simulink model "mech_car_handling"  (Simulink 7.1)
settings: Solver=ode15s  StartTime=0.0  StopTime=150  RelTol=1e-3
PostLoadFcn:
  | %%%%%%%%%%%%%%%%%%%%%%%%%%%%%%%%%%%%%%%%%%%%%%%%%%%%%%%%%%%%%%%%%%%%%%%%%%%
  | % INITIALIZE VEHICLE PARAMETERS
  | %%%%%%%%%%%%%%%%%%%%%%%%%%%%%%%%%%%%%%%%%%%%%%%%%%%%%%%%%%%%%%%%%%%%%%%%%%%
  | %clear;
  | %echo on;
  | 
  | % INITIALIZE STRUCTURES
  | chassis = struct();
  | wheel = struct();
  | axle = struct();
  | 
  | % INITIALIZE CHASSIS PARAMETERS
  | chassis.a = 1.50;          % longitudinal distance from CG to front axle
  | chassis.b = 0.99;           % longitudinal distance from CG to rear axle
  | chassis.w = 0.9;           % chassis width (wheel to wheel distance)
  | chassis.hu = 0.1;          % height of unsprung mass above ground
  | chassis.hs = 0.3;          % height of sprung mass above unsprung mass
  | chassis.ms = 1470;      % mass of sprung mass
  | chassis.mu = 200;        % mass of unsprung mass
  | 
  | % INITIALIZE WHEEL PARAMETERS
  | wheel.r = 0.3;             % wheel radius
  | wheel.m = 30;            % wheel mass
  | wheel.I = [0.52 0 0;0 1 0;0 0 0.52];
  | 
  | % INITIALIZE AXLE PARAMETERS
  | axle.m = 2;                 % axle mass
  | 
  | % COMPUTE STEADY STATE LOADS
  | Fzf = 0.5*(chassis.ms+chassis.mu) * 9.81 * chassis.b / (chassis.a + chassis.b);    % initial front wheel reaction
  | Fzr = 0.5*(chassis.ms+chassis.mu) * 9.81 * chassis. a / (chassis.a + chassis.b);    % initial rear wheel reaction
  | 
  | % INITIALIZE ROLL PARAMETERS
  | kf = 9000;                 % sprung front roll stiffness
  | kb = 5500;                % sprung rear roll stiffness
  | ku = 10000;              % unsprung roll stiffness (same front and rear)
  | bu = 0.1 * ku;            % unsprung roll damping
  | kr = kf + kb;              % total sprung roll stiffness
  | br = 0.1*kr;                % sprung roll damping
  | 
  | % INITIALIZE NONLINEAR TIRE MODEL PARAMETERS
  | a1 = 1.8658e-5;            % nonlinear tire model proportional coefficient
  | a2 = 9.3290e-4;            % nonlinear tire model quadratic coefficient
  | 
  | % INITIALIZE CONTROLLER PARAMETERS
  | Kp = 10000;                 % speed controller proportional gain
  | 
  | % INITIALIZE STEERING PARAMETERS
  | steeringAngle = 2;
  | %echo off;
StopFcn:
  | appDataName = 'mech_car_steering_fig_data';
  | mech_car_handling_fig_mgr('init',appDataName);
  | 
  | p = size(speed.signals.values);
  | p = p(1);
  | R = speed.signals.values([30:p])./yaw_rate.signals.values([30:p]);
  | modelFigure = getappdata(0,'mech_car_steering_fig_data');
  | plot(speed.signals.values([30:p]),R,'g','Parent',modelFigure.axesH);
libraries: mblibv1 x33, simulink x3
(part 1 of 2)
Description:
  | Car Handling
  | 
  | This model simulates the handling of a car for a set of chassis, wheel and axle characteristics. You can simulate the model for one roll stiffness, or for a range of roll stiffnesses by clicking on the blue subsystem.
  | 
  | The model shows that when a car is accelerated at a constant steering angle, it circles either out or in, depending on whether the car is understeered or oversteered, respectively.
CloseFcn:
  | appDataName = 'mech_car_steering_fig_data';
  | mech_car_handling_fig_mgr('destroy',appDataName);
settings Model: Creator=arnav  LastModifiedBy=batserve  ExtModeAutoUpdateStatusClock=off
settings DebuggingCC: SaveWithParameterizedLinksMsg=none  SignalResolutionControl=TryResolveAllWithWarning  SolverPrmCheckMsg=none  MultiTaskDSMMsg=warning  MultiTaskCondExecSysMsg=none  StrictBusMsg=None
settings HardwareCC: TargetBitPerLong=64  TargetEndianess=LittleEndian  TargetWordSize=64  TargetHWDeviceType=MATLAB Host  ProdEqTarget=off
settings RTWCC: SystemTargetFile=rsim.tlc  TemplateMakefile=rsim_default_tmf  Description=Rapid Simulation Target  ProcessScript=rsim_make_rtw_hook  IncludeERTFirstTime=on
settings RSimTargetCC: TargetFcnLib=ansi_tfl_tmw.mat  TargetFunctionLibrary=ANSI_C  IsPILTarget=off  EnableShiftOperators=on  PortableWordSizes=off
settings SimMechanicsCC: WarnOnRedundantConstraints=off

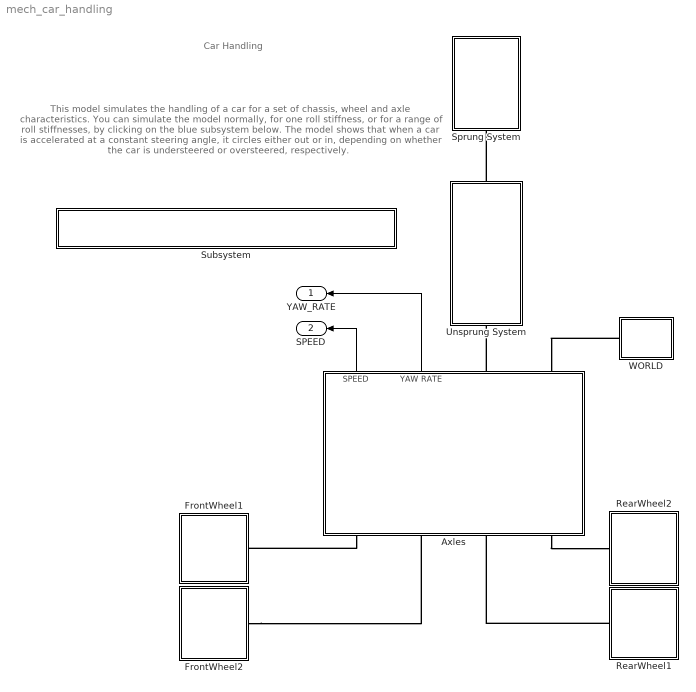
== system mech_car_handling ==
  note: Car Handling
  note: This model simulates the handling of a car for
      | a set of chassis, wheel and axle characteristics.
      | You can simulate the model normally, for one roll stiffness, or
      | for a range of roll stiffnesses, by clicking on the blue subsystem below.
      |
      | The model shows that when a car is accelerated at a constant steering
      | angle, it circles either out or in, depending on whether
      | the car is understeered or oversteered, respectively.
  Axles : Subsystem  Orientation=up  mask{w=chassis.w, a=chassis.a, b=chassis.b, m=axle.m}
      mask prompts: w "Axle Length"; a "CG to Front Axle Distance"; b "CG to Rear Axle Distance"; m "Axle Mass"
      mask Display: image(imread('double_wishbone.jpg'))
  FrontWheel1 : Subsystem  Orientation=left
      mask Display: image(imread('wheel.jpg'))
  FrontWheel2 : Subsystem  Orientation=left
      mask Display: image(imread('wheel.jpg'))
  RearWheel1 : Subsystem
      mask Display: image(imread('wheel.jpg'))
  RearWheel2 : Subsystem
      mask Display: image(imread('wheel.jpg'))
  Sprung System : Subsystem  Orientation=up
  Subsystem : Subsystem
      settings: OpenFcn=mech_car_handling_sweep
      mask Display: disp('CLICK HERE TO RUN FOR A RANGE OF ROLL STIFFNESSES')
  Unsprung System : Subsystem  Orientation=up
  WORLD : Subsystem
      mask Display: image(imread('sky.jpg'))
  YAW_RATE : Outport  Orientation=left  OutDataType=sfix(16)  OutScaling=2^0
  SPEED : Outport  Orientation=left  Port=2  OutDataType=sfix(16)  OutScaling=2^0
  wires:
  Axles/1(SPEED) -> SPEED/1
  Axles/2(YAW RATE) -> YAW_RATE/1
  connections:
  WORLD/LConn1 -- Axles/RConn2
  FrontWheel2/LConn1 -- Axles/LConn2
  RearWheel1/LConn1 -- Axles/LConn3
  Axles/LConn4 -- RearWheel2/LConn1
  Axles/LConn1 -- FrontWheel1/LConn1
  Axles/RConn1 -- Unsprung System/LConn1
  Unsprung System/RConn1 -- Sprung System/LConn1

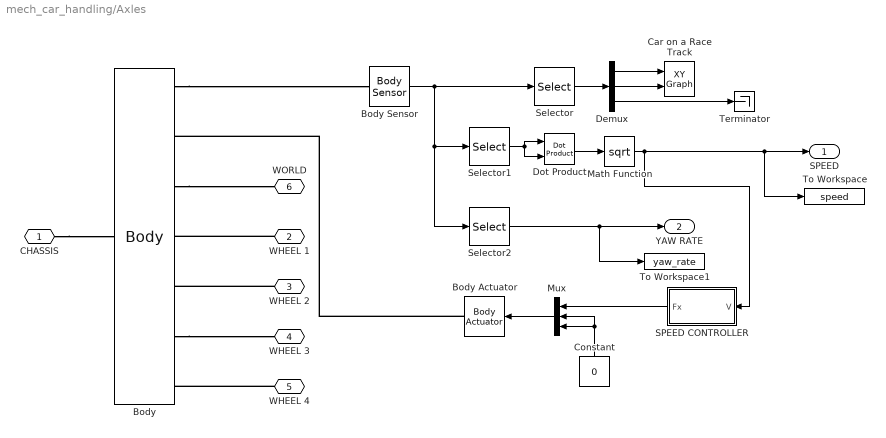
== system mech_car_handling/Axles ==
  Body : mblibv1/Bodies/Body  DialogController=MECH.DynMechDlgSource  PhysicalDomain=mechanical  SubClassName=Unknown  LeftPortType=workingframe  RightPortType=workingframe  LConnTagsString=CG  RConnTagsString=CS6|CS7|CS3|CS1|CS2|CS4|CS5  DialogClass=MechanicalBodyBlock  Mass=2*m  MassUnits=kg  InertiaUnits=kg*m^2  Inertia=[0.12 0 0; 0 1.5 0;0 0 1.5]  Shape=Cylinder  ShapeDims=[1 1]  ShapeUnits=m  ShapeUse=false  Density=1  DensityUnits=kg/m^3  DensityUse=false  GraphicsMode=1  BodyColor=[0.5 0.5 0.5]  GraphicsObj=[]  AttachedToCS=1  CG=Left$CG$[0 0 0]$CS3$CS3$m$[0 0 0]$EULER X-Y-Z$deg$WORLD$true  WorkingFrames=Right$CS6$[0 0 0]$CS3$CS3$m$[0 0 0]$EULER X-Y-Z$deg$WORLD$true#Right$CS7$[0 0 0]$CS3$CS3$m$[0 0 0]$EULER X-Y-Z$deg$WORLD$true#Right$CS3$[0 0 0]$ADJOINING$ADJOINING$m$[0 0 0]$EULER X-Y-Z$deg$WORLD$true#Right$CS1$[a -0.5*w 0]$CS3$CS3$m$[0 0 0]$EULER X-Y-Z$deg$WORLD$true#Right$CS2$[a 0.5*w 0]$CS3$CS3$m$[0 0 0]$EULER X-Y-Z$deg$WORLD$true#Right$CS4$[-b -0.5*w 0]$CS3$CS3$m$[0 0 0]$EULER X-Y-Z$deg$WORLD$true#Right$CS5$[-b 0.5*w 0]$CS3$CS3$m$[0 0 0]$EULER X-Y-Z$deg$WORLD$true  CGPos=[0 0 0]  CGRot=[0 0 0]  CS0Pos=[]  CS0Rot=[]  CS1Pos=[a -0.5*w 0]  CS1Rot=[0 0 0]  CS2Pos=[a 0.5*w 0]  CS2Rot=[0 0 0]  CS3Pos=[0 0 0]  CS3Rot=[0 0 0]  CS4Pos=[-b -0.5*w 0]  CS4Rot=[0 0 0]  CS5Pos=[-b 0.5*w 0]  CS5Rot=[0 0 0]  CS6Pos=[0 0 0]  CS6Rot=[0 0 0]  CS7Pos=[0 0 0]  CS7Rot=[0 0 0]  CS8Pos=[]  CS8Rot=[]  CS9Pos=[]  CS9Rot=[]  CS10Pos=[]  CS10Rot=[]  CS11Pos=[]  CS11Rot=[]  CS12Pos=[]  CS12Rot=[]  CS13Pos=[]  CS13Rot=[]  CS14Pos=[]  CS14Rot=[]  CS15Pos=[]  CS15Rot=[]  CS16Pos=[]  CS16Rot=[]  CS17Pos=[]  CS17Rot=[]  CS18Pos=[]  CS18Rot=[]  CS19Pos=[]  CS19Rot=[]  CS20Pos=[]  CS20Rot=[]
  Body Actuator : mblibv1/Sensors &  Actuators/Body Actuator  Orientation=left  DialogController=MECH.DynMechDlgSource  SystemSampleTime=-1  PhysicalDomain=Mechanical  PortType=blob  ActuationStyle=Force  AngleUnits=deg  ArcVelocityUnits=deg/s  ArcAccelerationUnits=deg/s^2  CoordPositionUnits=m  VelocityUnits=m/s  AccelerationUnits=m/s^2  ForceUnits=N  TorqueUnits=N-m  ActiveIO=on  Width=3  DialogClass=MechanicalActuatorBlock  ReferenceFrame=Local (Body CS)  Angle=off  CoordPosition=on  Force=on  Torque=off
  Body Sensor : mblibv1/Sensors &  Actuators/Body Sensor  DialogController=MECH.DynMechDlgSource  SystemSampleTime=-1  PhysicalDomain=Mechanical  PortType=blob  Muxed=on  Pose=off  Angle=on  AngleUnits=deg  ArcVelocity=on  ArcVelocityUnits=rad/s  ArcAcceleration=off  ArcAccelerationUnits=deg/s^2  CoordPosition=on  CoordPositionUnits=m  Velocity=on  VelocityUnits=m/s  Acceleration=off  AccelerationUnits=m/s^2  Quaternion=on  QuaternionDT=off  QuaternionDDT=off  QuaternionUnits=off  OutputVector=[ 3 3 3 ]  ActiveIO=on  Width=9  DialogClass=MechanicalSensorBlock  ReferenceFrame=Absolute (World)
  Car on a Race Track : simulink/Sinks/XY Graph  SystemSampleTime=-1  xmin=-200  xmax=200  ymin=-100  ymax=250  st=-1
  Constant : Constant  Orientation=up  Value=0  OutDataType=sfix(16)  OutScaling=2^0
  Demux : Demux  Outputs=3
  Dot Product : simulink/Math Operations/Dot Product  InputSameDT=on  OutDataType=sfix(16)  OutScaling=2^-10  DoSatur=off
  Math Function : Math  Operator=sqrt  OutDataType=sfix(16)  OutScaling=2^0  SaturateOnIntegerOverflow=on
  Mux : Mux  Orientation=left  Inputs=3
  SPEED CONTROLLER : Subsystem  Orientation=left
  Selector : Selector  InputPortWidth=9  IndexOptions=Index vector (dialog)  Indices=[1 2 3]  OutputSizes=1
  Selector1 : Selector  InputPortWidth=9  IndexOptions=Index vector (dialog)  Indices=[4 5]  OutputSizes=1
  Selector2 : Selector  InputPortWidth=9  IndexOptions=Index vector (dialog)  Indices=9  OutputSizes=1
  Terminator : Terminator
  To Workspace : ToWorkspace  VariableName=speed  SampleTime=-1  SaveFormat=Structure
  To Workspace1 : ToWorkspace  VariableName=yaw_rate  SampleTime=-1  SaveFormat=Structure
  CHASSIS : PMIOPort  Port=1  Side=Right
  WHEEL 1 : PMIOPort  Orientation=left  Port=2  Side=Left
  WHEEL 2 : PMIOPort  Orientation=left  Port=3  Side=Left
  WHEEL 3 : PMIOPort  Orientation=left  Port=4  Side=Left
  WHEEL 4 : PMIOPort  Orientation=left  Port=5  Side=Left
  WORLD : PMIOPort  Orientation=left  Port=6  Side=Right
  SPEED : Outport  OutDataType=sfix(16)  OutScaling=2^0
  YAW RATE : Outport  Port=2  OutDataType=sfix(16)  OutScaling=2^0
  wires:
  Demux/1 -> Car on a Race Track/1
  Demux/2 -> Car on a Race Track/2
  Dot Product/1 -> Math Function/1
  Math Function/1 -> SPEED CONTROLLER/1(V), SPEED/1, To Workspace/1
  Selector/1 -> Demux/1
  Body Sensor/1 -> Selector/1, Selector1/1, Selector2/1
  Selector1/1 -> Dot Product/1, Dot Product/2
  Selector2/1 -> YAW RATE/1, To Workspace1/1
  Constant/1 -> Mux/3, Mux/2
  Mux/1 -> Body Actuator/1
  SPEED CONTROLLER/1(Fx) -> Mux/1
  Demux/3 -> Terminator/1
  connections:
  WHEEL 1/RConn1 -- Body/RConn4
  CHASSIS/RConn1 -- Body/LConn1
  WHEEL 2/RConn1 -- Body/RConn5
  Body/RConn3 -- WORLD/RConn1
  WHEEL 4/RConn1 -- Body/RConn7
  Body/RConn6 -- WHEEL 3/RConn1
  Body/RConn1 -- Body Sensor/LConn1
  Body Actuator/RConn1 -- Body/RConn2

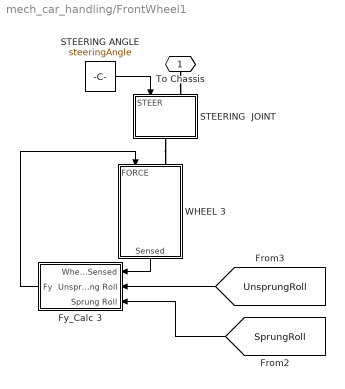
== system mech_car_handling/FrontWheel1 ==
  Fy_Calc 3 : Subsystem  Orientation=left
  STEERING ANGLE : Constant  Value=steeringAngle  OutDataType=sfix(16)  OutScaling=2^0
  STEERING  JOINT : Subsystem  Orientation=down
  WHEEL 3 : Subsystem  Orientation=down  mask{r=wheel.r, m=wheel.m, I=wheel.I}
      mask prompts: r "Wheel Radius"; m "Wheel Mass"; I "Wheel Inertia"
  To Chassis : PMIOPort  Orientation=down  Port=1  Side=Left
  wires:
  STEERING ANGLE/1 -> STEERING  JOINT/1(STEER)
  Fy_Calc 3/1(Fy) -> WHEEL 3/1(FORCE)
  WHEEL 3/1(Sensed) -> Fy_Calc 3/1(Wheel Sensed)
  [UnsprungRoll] -> Fy_Calc 3/2(Unsprung Roll)
  [SprungRoll] -> Fy_Calc 3/3(Sprung Roll)
  connections:
  STEERING  JOINT/RConn1 -- WHEEL 3/LConn1
  To Chassis/RConn1 -- STEERING  JOINT/LConn1

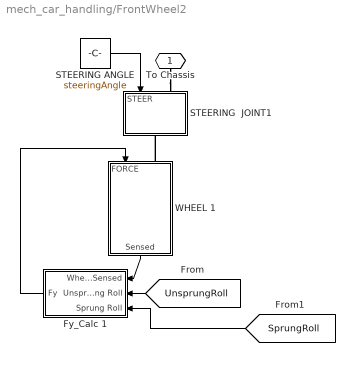
== system mech_car_handling/FrontWheel2 ==
  Fy_Calc 1 : Subsystem  Orientation=left
  STEERING ANGLE : Constant  Value=steeringAngle  OutDataType=sfix(16)  OutScaling=2^0
  STEERING  JOINT1 : Subsystem  Orientation=down
  WHEEL 1 : Subsystem  Orientation=down  mask{r=wheel.r, m=wheel.m, I=wheel.I}
      mask prompts: r "Wheel Radius"; m "Wheel Mass"; I "Wheel Inertia"
  To Chassis : PMIOPort  Orientation=down  Port=1  Side=Left
  wires:
  WHEEL 1/1(Sensed) -> Fy_Calc 1/1(Wheel Sensed)
  [UnsprungRoll] -> Fy_Calc 1/2(Unsprung Roll)
  [SprungRoll] -> Fy_Calc 1/3(Sprung Roll)
  STEERING ANGLE/1 -> STEERING  JOINT1/1(STEER)
  Fy_Calc 1/1(Fy) -> WHEEL 1/1(FORCE)
  connections:
  WHEEL 1/LConn1 -- STEERING  JOINT1/RConn1
  To Chassis/RConn1 -- STEERING  JOINT1/LConn1

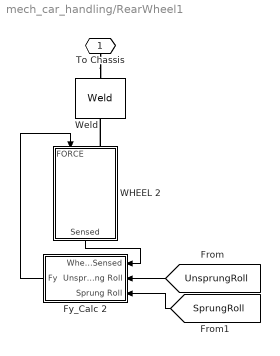
== system mech_car_handling/RearWheel1 ==
  Fy_Calc 2 : Subsystem  Orientation=left
  WHEEL 2 : Subsystem  Orientation=down  mask{r=wheel.r, m=wheel.m, I=wheel.I}
      mask prompts: r "Wheel Radius"; m "Wheel Mass"; I "Wheel Inertia"
  Weld : mblibv1/Joints/Weld  Orientation=down  DialogController=MECH.DynMechDlgSource  PhysicalDomain=mechanical  SubClassName=Unknown  LeftPortType=blob  RightPortType=blob  LConnTagsString=__newl0  RConnTagsString=__newr0  NumSAPorts=0  CutJoint=off  MarkAsCut=off  Primitives=weld  PrimitiveProps=W$INERTIAL$[0 0 0]$weld  DialogClass=JointBlock  WAxis=[0 0 0]
  To Chassis : PMIOPort  Orientation=down  Port=1  Side=Left
  wires:
  Fy_Calc 2/1(Fy) -> WHEEL 2/1(FORCE)
  WHEEL 2/1(Sensed) -> Fy_Calc 2/1(Wheel Sensed)
  [UnsprungRoll] -> Fy_Calc 2/2(Unsprung Roll)
  [SprungRoll] -> Fy_Calc 2/3(Sprung Roll)
  connections:
  WHEEL 2/LConn1 -- Weld/RConn1
  To Chassis/RConn1 -- Weld/LConn1

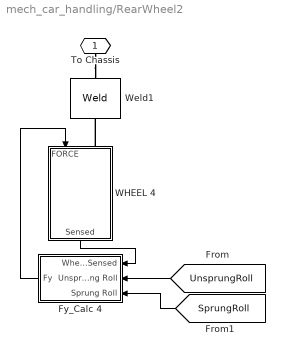
== system mech_car_handling/RearWheel2 ==
  Fy_Calc 4 : Subsystem  Orientation=left
  WHEEL 4 : Subsystem  Orientation=down  mask{r=wheel.r, m=wheel.m, I=wheel.I}
      mask prompts: r "Wheel Radius"; m "Wheel Mass"; I "Wheel Inertia"
  Weld1 : mblibv1/Joints/Weld  Orientation=down  DialogController=MECH.DynMechDlgSource  PhysicalDomain=mechanical  SubClassName=Unknown  LeftPortType=blob  RightPortType=blob  LConnTagsString=__newl0  RConnTagsString=__newr0  NumSAPorts=0  CutJoint=off  MarkAsCut=off  Primitives=weld  PrimitiveProps=W$INERTIAL$[0 0 0]$weld  DialogClass=JointBlock  WAxis=[0 0 0]
  To Chassis : PMIOPort  Orientation=down  Port=1  Side=Left
  wires:
  Fy_Calc 4/1(Fy) -> WHEEL 4/1(FORCE)
  WHEEL 4/1(Sensed) -> Fy_Calc 4/1(Wheel Sensed)
  [UnsprungRoll] -> Fy_Calc 4/2(Unsprung Roll)
  [SprungRoll] -> Fy_Calc 4/3(Sprung Roll)
  connections:
  WHEEL 4/LConn1 -- Weld1/RConn1
  To Chassis/RConn1 -- Weld1/LConn1

== system mech_car_handling/Sprung System ==
  note: Sprung mass represents the
      | total mass of the car: the mass
      | of the wheels and chassis.
  SPRUNG MASS : Subsystem  Orientation=down  mask{a=chassis.a, b=chassis.b, m=chassis.ms, h=chassis.hs}
      mask prompts: a "Front Axle to CG Distance"; b "Rear Axle to CG Distance"; m "Chassis Mass"; h "CG Height (above axles)"
  TORSIONAL SPRING1 : Subsystem  Orientation=up
  To UnSprungMass : PMIOPort  Orientation=up  Port=1  Side=Left
  tag scope: SprungRoll=global
  wires:
  TORSIONAL SPRING1/1(Roll) -> [SprungRoll]
  connections:
  TORSIONAL SPRING1/RConn1 -- SPRUNG MASS/RConn1
  To UnSprungMass/RConn1 -- TORSIONAL SPRING1/LConn1

== system mech_car_handling/Subsystem ==

== system mech_car_handling/Unsprung System ==
  note: Sprung mass represents the
      | the mass of the wheels and
      | chassis only.
  TORSIONAL SPRING : Subsystem  Orientation=up
  UNSPRUNG MASS : Subsystem  Orientation=down  mask{a=chassis.a, b=chassis.b, m=chassis.mu, h=chassis.hu}
      mask prompts: a "Front Axle to CG Distance"; b "Rear Axle to CG Distance"; m "Chassis Mass"; h "CG Height (above axles)"
  To SprungSystem : PMIOPort  Orientation=down  Port=1  Side=Right
  To Chassis : PMIOPort  Orientation=up  Port=2  Side=Left
  tag scope: UnsprungRoll=global
  wires:
  TORSIONAL SPRING/1(Roll) -> [UnsprungRoll]
  connections:
  TORSIONAL SPRING/RConn1 -- UNSPRUNG MASS/RConn1
  To SprungSystem/RConn1 -- UNSPRUNG MASS/LConn1
  To Chassis/RConn1 -- TORSIONAL SPRING/LConn1

== system mech_car_handling/WORLD ==
  Ground : mblibv1/Bodies/Ground  Orientation=left  DialogController=MECH.DynMechDlgSource  SystemSampleTime=-1  LeftPortType=env  RightPortType=workingframe  PhysicalDomain=Mechanical  DialogClass=GroundBlock  CoordPosition=[0 0 0]  CoordPositionUnits=m  StateVectorMgrId=-1  MachineId=[0 0]  ShowEnvPort=on
  Joint Initial Condition : mblibv1/Sensors &  Actuators/Joint Initial Condition  DialogController=MECH.DynMechDlgSource  SystemSampleTime=-1  PhysicalDomain=mechanical  DialogClass=InitialConditionBlock  InitialConditions=P1$true$0$m$rad$2$m/s$rad/s#P2$true$0$m$rad$0$m/s$rad/s#P3$false$0$m$rad$0$m/s$rad/s#R1$false$0$m$rad$0$m/s$rad/s#R2$false$0$m$rad$0$m/s$rad/s#R3$false$0$m$rad$0$m/s$rad/s#S$false$0$m$rad$0$m/s$rad/s  P1PIC=0  P1VIC=2  P2PIC=0  P2VIC=0  P3PIC=0  P3VIC=0  R1PIC=0  R1VIC=0  R2PIC=0  R2VIC=0  R3PIC=0  R3VIC=0  SPIC=0  SVIC=0
  Machine Environment : mblibv1/Bodies/Machine Environment  Tag=Factory ground  Orientation=left  DialogController=MECH.DialogSource  SystemSampleTime=-1  PortType=env  PhysicalDomain=Mechanical  DialogTemplateClass=MECH.MachineEnvironment  SyncWhenCopied=off  Gravity=[0 0 -9.81]  GravityUnits=m/s^2  GravityAsSignal=off  Dimensionality=Auto-detect  AnalysisType=Forward dynamics  LinearAssemblyTolerance=1e-3  LinearAssemblyToleranceUnits=m  AngularAssemblyTolerance=1e-3  AngularAssemblyToleranceUnits=rad  ConstraintSolverType=Stabilizing  ConstraintRelTolerance=1e-4  ConstraintAbsTolerance=1e-4  UseRobustSingularityHandling=off  RedundancyAnalysisToleranceType=Automatically select tolerance  RedundancyAnalysisTolerance=1e-14  StatePerturbationType=Fixed  PerturbationSize=1e-5  VisualizeMachine=on
  Planar : mblibv1/Joints/Planar  Orientation=left  DialogController=MECH.DynMechDlgSource  PhysicalDomain=mechanical  SubClassName=Unknown  LeftPortType=blob  RightPortType=blob  LConnTagsString=__newl0|SA1  RConnTagsString=__newr0  NumSAPorts=1  CutJoint=off  MarkAsCut=off  Primitives=prismatic_prismatic_revolute  PrimitiveProps=P1$WORLD$[1 0 0]$prismatic#P2$WORLD$[0 1 0]$prismatic#R1$WORLD$[0 0 1]$revolute  DialogClass=JointBlock  P1Axis=[1 0 0]  P2Axis=[0 1 0]  R1Axis=[0 0 1]
  F : PMIOPort  Port=1  Side=Left
  connections:
  Machine Environment/RConn1 -- Ground/LConn1
  F/RConn1 -- Planar/RConn1
  Ground/RConn1 -- Planar/LConn1
  Joint Initial Condition/RConn1 -- Planar/LConn2

== system mech_car_handling/Axles/SPEED CONTROLLER ==
  V : Inport  OutDataType=sfix(16)  OutScaling=2^0
  Kp : Gain  Gain=Kp  ParameterDataType=sfix(16)  ParameterScaling=2^0  OutDataType=sfix(16)  OutScaling=2^0
  Kp1 : Gain  Gain=-1  ParameterDataType=sfix(16)  ParameterScaling=2^0  OutDataType=sfix(16)  OutScaling=2^0
  Ramp : simulink/Sources/Ramp  SystemSampleTime=-1  slope=0.1  start=0  X0=5
  Subtract2 : Sum  Inputs=+-  OutDataType=sfix(16)  OutScaling=2^-10
  Fx : Outport  OutDataType=sfix(16)  OutScaling=2^0
  wires:
  V/1 -> Subtract2/1
  Subtract2/1 -> Kp/1
  Ramp/1 -> Subtract2/2
  Kp1/1 -> Fx/1
  Kp/1 -> Kp1/1

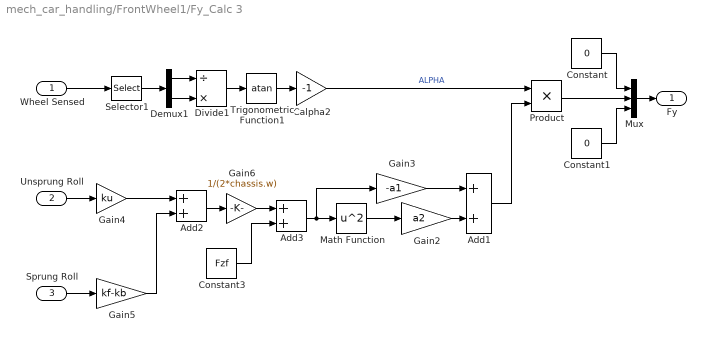
== system mech_car_handling/FrontWheel1/Fy_Calc 3 ==
  Wheel Sensed : Inport  OutDataType=sfix(16)  OutScaling=2^0
  Unsprung Roll : Inport  Port=2  OutDataType=sfix(16)  OutScaling=2^0
  Sprung Roll : Inport  Port=3  OutDataType=sfix(16)  OutScaling=2^0
  Add1 : Sum  OutDataType=sfix(16)  OutScaling=2^-10
  Add2 : Sum  OutDataType=sfix(16)  OutScaling=2^-10
  Add3 : Sum  OutDataType=sfix(16)  OutScaling=2^-10
  Calpha2 : Gain  Gain=-1  ParameterDataType=sfix(16)  ParameterScaling=2^0  OutDataType=sfix(16)  OutScaling=2^0
  Constant : Constant  Value=0  OutDataType=sfix(16)  OutScaling=2^0
  Constant1 : Constant  Value=0  OutDataType=sfix(16)  OutScaling=2^0
  Constant3 : Constant  Value=Fzf  OutDataType=sfix(16)  OutScaling=2^0
  Demux1 : Demux  Outputs=2
  Divide1 : Product  Inputs=/*  OutDataType=sfix(16)  OutScaling=2^-10
  Gain2 : Gain  Gain=a2  ParameterDataType=sfix(16)  ParameterScaling=2^0  OutDataType=sfix(16)  OutScaling=2^0
  Gain3 : Gain  Gain=-a1  ParameterDataType=sfix(16)  ParameterScaling=2^0  OutDataType=sfix(16)  OutScaling=2^0
  Gain4 : Gain  Gain=ku  ParameterDataType=sfix(16)  ParameterScaling=2^0  OutDataType=sfix(16)  OutScaling=2^0
  Gain5 : Gain  Gain=kf-kb  ParameterDataType=sfix(16)  ParameterScaling=2^0  OutDataType=sfix(16)  OutScaling=2^0
  Gain6 : Gain  Gain=1/(2*chassis.w)  ParameterDataType=sfix(16)  ParameterScaling=2^0  OutDataType=sfix(16)  OutScaling=2^0
  Math Function : Math  Operator=square  OutDataType=sfix(16)  OutScaling=2^0  SaturateOnIntegerOverflow=on
  Mux : Mux  Inputs=3
  Product : Product  OutDataType=sfix(16)  OutScaling=2^0  RndMeth=Zero
  Selector1 : Selector  InputPortWidth=3  IndexOptions=Index vector (dialog)  Indices=[1 2]  OutputSizes=1
  Trigonometric Function1 : Trigonometry  Operator=atan
  Fy : Outport  OutDataType=sfix(16)  OutScaling=2^0
  wires:
  Calpha2/1 -> Product/1  "ALPHA"
  Divide1/1 -> Trigonometric Function1/1
  Demux1/2 -> Divide1/2
  Demux1/1 -> Divide1/1
  Selector1/1 -> Demux1/1
  Constant1/1 -> Mux/3
  Constant/1 -> Mux/1
  Mux/1 -> Fy/1
  Product/1 -> Mux/2
  Wheel Sensed/1 -> Selector1/1
  Trigonometric Function1/1 -> Calpha2/1
  Math Function/1 -> Gain2/1
  Gain2/1 -> Add1/2
  Gain3/1 -> Add1/1
  Add1/1 -> Product/2
  Unsprung Roll/1 -> Gain4/1
  Sprung Roll/1 -> Gain5/1
  Gain4/1 -> Add2/1
  Gain5/1 -> Add2/2
  Add2/1 -> Gain6/1
  Gain6/1 -> Add3/1
  Constant3/1 -> Add3/2
  Add3/1 -> Math Function/1, Gain3/1

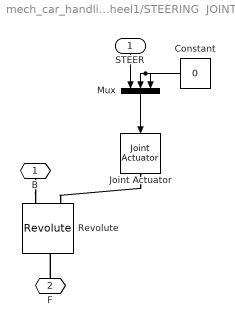
== system mech_car_handling/FrontWheel1/STEERING  JOINT ==
  STEER : Inport  Orientation=down  OutDataType=sfix(16)  OutScaling=2^0
  Constant : Constant  Orientation=left  Value=0  OutDataType=sfix(16)  OutScaling=2^0
  Joint Actuator : mblibv1/Sensors &  Actuators/Joint Actuator  Orientation=down  DialogController=MECH.DynMechDlgSource  SystemSampleTime=-1  PhysicalDomain=Mechanical  PortType=blob  ActuationStyle=Motion  AngleUnits=deg  ArcVelocityUnits=deg/s  ArcAccelerationUnits=deg/s^2  CoordPositionUnits=m  VelocityUnits=m/s  AccelerationUnits=m/s^2  ForceUnits=N  TorqueUnits=N-m  ActiveIO=on  Width=3  DialogClass=MechanicalActuatorBlock  Primitive=R1  ReferenceFrame=Absolute (INERTIAL)
  Mux : Mux  Orientation=down  Inputs=3
  Revolute : mblibv1/Joints/Revolute  Orientation=down  DialogController=MECH.DynMechDlgSource  PhysicalDomain=mechanical  SubClassName=Unknown  LeftPortType=blob  RightPortType=blob  LConnTagsString=__newl0|SA1  RConnTagsString=__newr0  NumSAPorts=1  CutJoint=off  MarkAsCut=off  Primitives=revolute  PrimitiveProps=R1$WORLD$[0 0 1]$revolute  DialogClass=JointBlock  R1Axis=[0 0 1]
  B : PMIOPort  Orientation=down  Port=1  Side=Left
  F : PMIOPort  Orientation=up  Port=2  Side=Right
  wires:
  STEER/1 -> Mux/1
  Mux/1 -> Joint Actuator/1
  Constant/1 -> Mux/2, Mux/3
  connections:
  Joint Actuator/RConn1 -- Revolute/LConn2
  B/RConn1 -- Revolute/LConn1
  F/RConn1 -- Revolute/RConn1

== system mech_car_handling/FrontWheel1/WHEEL 3 ==
  FORCE : Inport  Orientation=left  OutDataType=sfix(16)  OutScaling=2^0
  Body : mblibv1/Bodies/Body  DialogController=MECH.DynMechDlgSource  PhysicalDomain=mechanical  SubClassName=Unknown  LeftPortType=workingframe  RightPortType=workingframe  LConnTagsString=CG  RConnTagsString=CS2|CS3  DialogClass=MechanicalBodyBlock  Mass=m  MassUnits=kg  InertiaUnits=kg*m^2  Inertia=I  Shape=Cylinder  ShapeDims=[1 1]  ShapeUnits=m  ShapeUse=false  Density=1  DensityUnits=kg/m^3  DensityUse=false  GraphicsMode=1  BodyColor=[0.5 0.5 0.5]  GraphicsObj=[]  AttachedToCS=1  CG=Left$CG$[0 0 0]$ADJOINING$ADJOINING$m$[0 0 0]$EULER X-Y-Z$deg$WORLD$true  WorkingFrames=Right$CS2$[0 0 -r]$CG$CG$m$[0 0 0]$EULER X-Y-Z$deg$WORLD$true#Left$CS1$[0 0 -r]$CG$CG$m$[0 0 0]$EULER X-Y-Z$deg$WORLD$false#Right$CS3$[0 0 -r]$CG$CG$m$[0 0 0]$EULER X-Y-Z$deg$WORLD$true  CGPos=[0 0 0]  CGRot=[0 0 0]  CS0Pos=[]  CS0Rot=[]  CS1Pos=[0 0 -r]  CS1Rot=[0 0 0]  CS2Pos=[0 0 -r]  CS2Rot=[0 0 0]  CS3Pos=[0 0 -r]  CS3Rot=[0 0 0]  CS4Pos=[]  CS4Rot=[]  CS5Pos=[]  CS5Rot=[]  CS6Pos=[]  CS6Rot=[]  CS7Pos=[]  CS7Rot=[]  CS8Pos=[]  CS8Rot=[]  CS9Pos=[]  CS9Rot=[]  CS10Pos=[]  CS10Rot=[]  CS11Pos=[]  CS11Rot=[]  CS12Pos=[]  CS12Rot=[]  CS13Pos=[]  CS13Rot=[]  CS14Pos=[]  CS14Rot=[]  CS15Pos=[]  CS15Rot=[]  CS16Pos=[]  CS16Rot=[]  CS17Pos=[]  CS17Rot=[]  CS18Pos=[]  CS18Rot=[]  CS19Pos=[]  CS19Rot=[]  CS20Pos=[]  CS20Rot=[]
  Body Actuator : mblibv1/Sensors &  Actuators/Body Actuator  Orientation=left  DialogController=MECH.DynMechDlgSource  SystemSampleTime=-1  PhysicalDomain=Mechanical  PortType=blob  ActuationStyle=Force  AngleUnits=deg  ArcVelocityUnits=deg/s  ArcAccelerationUnits=deg/s^2  CoordPositionUnits=m  VelocityUnits=m/s  AccelerationUnits=m/s^2  ForceUnits=N  TorqueUnits=N-m  ActiveIO=on  Width=3  DialogClass=MechanicalActuatorBlock  ReferenceFrame=Local (Body CS)  Angle=off  CoordPosition=on  Force=on  Torque=off
  Body Sensor : mblibv1/Sensors &  Actuators/Body Sensor  DialogController=MECH.DynMechDlgSource  SystemSampleTime=-1  PhysicalDomain=Mechanical  PortType=blob  Muxed=on  Pose=off  Angle=on  AngleUnits=deg  ArcVelocity=off  ArcVelocityUnits=deg/s  ArcAcceleration=off  ArcAccelerationUnits=deg/s^2  CoordPosition=off  CoordPositionUnits=m  Velocity=on  VelocityUnits=m/s  Acceleration=off  AccelerationUnits=m/s^2  Quaternion=on  QuaternionDT=off  QuaternionDDT=off  QuaternionUnits=off  OutputVector=[ 3 ]  ActiveIO=on  Width=3  DialogClass=MechanicalSensorBlock  ReferenceFrame=Local (Body CS)
  TO AXLE : PMIOPort  Port=1  Side=Left
  Sensed : Outport  OutDataType=sfix(16)  OutScaling=2^0
  wires:
  Body Sensor/1 -> Sensed/1
  FORCE/1 -> Body Actuator/1
  connections:
  TO AXLE/RConn1 -- Body/LConn1
  Body/RConn1 -- Body Sensor/LConn1
  Body Actuator/RConn1 -- Body/RConn2

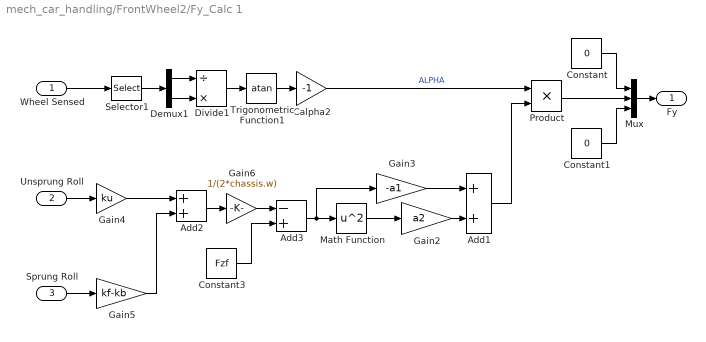
== system mech_car_handling/FrontWheel2/Fy_Calc 1 ==
  Wheel Sensed : Inport  OutDataType=sfix(16)  OutScaling=2^0
  Unsprung Roll : Inport  Port=2  OutDataType=sfix(16)  OutScaling=2^0
  Sprung Roll : Inport  Port=3  OutDataType=sfix(16)  OutScaling=2^0
  Add1 : Sum  OutDataType=sfix(16)  OutScaling=2^-10
  Add2 : Sum  OutDataType=sfix(16)  OutScaling=2^-10
  Add3 : Sum  Inputs=-+  OutDataType=sfix(16)  OutScaling=2^-10
  Calpha2 : Gain  Gain=-1  ParameterDataType=sfix(16)  ParameterScaling=2^0  OutDataType=sfix(16)  OutScaling=2^0
  Constant : Constant  Value=0  OutDataType=sfix(16)  OutScaling=2^0
  Constant1 : Constant  Value=0  OutDataType=sfix(16)  OutScaling=2^0
  Constant3 : Constant  Value=Fzf  OutDataType=sfix(16)  OutScaling=2^0
  Demux1 : Demux  Outputs=2
  Divide1 : Product  Inputs=/*  OutDataType=sfix(16)  OutScaling=2^-10
  Gain2 : Gain  Gain=a2  ParameterDataType=sfix(16)  ParameterScaling=2^0  OutDataType=sfix(16)  OutScaling=2^0
  Gain3 : Gain  Gain=-a1  ParameterDataType=sfix(16)  ParameterScaling=2^0  OutDataType=sfix(16)  OutScaling=2^0
  Gain4 : Gain  Gain=ku  ParameterDataType=sfix(16)  ParameterScaling=2^0  OutDataType=sfix(16)  OutScaling=2^0
  Gain5 : Gain  Gain=kf-kb  ParameterDataType=sfix(16)  ParameterScaling=2^0  OutDataType=sfix(16)  OutScaling=2^0
  Gain6 : Gain  Gain=1/(2*chassis.w)  ParameterDataType=sfix(16)  ParameterScaling=2^0  OutDataType=sfix(16)  OutScaling=2^0
  Math Function : Math  Operator=square  OutDataType=sfix(16)  OutScaling=2^0  SaturateOnIntegerOverflow=on
  Mux : Mux  Inputs=3
  Product : Product  OutDataType=sfix(16)  OutScaling=2^0  RndMeth=Zero
  Selector1 : Selector  InputPortWidth=3  IndexOptions=Index vector (dialog)  Indices=[1 2]  OutputSizes=1
  Trigonometric Function1 : Trigonometry  Operator=atan
  Fy : Outport  OutDataType=sfix(16)  OutScaling=2^0
  wires:
  Add3/1 -> Gain3/1, Math Function/1
  Constant3/1 -> Add3/2
  Gain6/1 -> Add3/1
  Add2/1 -> Gain6/1
  Gain5/1 -> Add2/2
  Gain4/1 -> Add2/1
  Sprung Roll/1 -> Gain5/1
  Unsprung Roll/1 -> Gain4/1
  Add1/1 -> Product/2
  Gain3/1 -> Add1/1
  Gain2/1 -> Add1/2
  Math Function/1 -> Gain2/1
  Trigonometric Function1/1 -> Calpha2/1
  Wheel Sensed/1 -> Selector1/1
  Product/1 -> Mux/2
  Mux/1 -> Fy/1
  Constant/1 -> Mux/1
  Constant1/1 -> Mux/3
  Selector1/1 -> Demux1/1
  Demux1/1 -> Divide1/1
  Demux1/2 -> Divide1/2
  Divide1/1 -> Trigonometric Function1/1
  Calpha2/1 -> Product/1  "ALPHA"

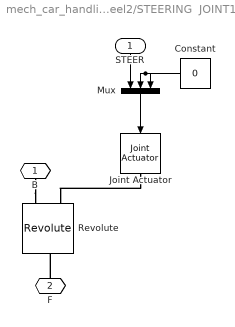
== system mech_car_handling/FrontWheel2/STEERING  JOINT1 ==
  STEER : Inport  Orientation=down  OutDataType=sfix(16)  OutScaling=2^0
  Constant : Constant  Orientation=left  Value=0  OutDataType=sfix(16)  OutScaling=2^0
  Joint Actuator : mblibv1/Sensors &  Actuators/Joint Actuator  Orientation=down  DialogController=MECH.DynMechDlgSource  SystemSampleTime=-1  PhysicalDomain=Mechanical  PortType=blob  ActuationStyle=Motion  AngleUnits=deg  ArcVelocityUnits=deg/s  ArcAccelerationUnits=deg/s^2  CoordPositionUnits=m  VelocityUnits=m/s  AccelerationUnits=m/s^2  ForceUnits=N  TorqueUnits=N-m  ActiveIO=on  Width=3  DialogClass=MechanicalActuatorBlock  Primitive=R1  ReferenceFrame=Absolute (INERTIAL)
  Mux : Mux  Orientation=down  Inputs=3
  Revolute : mblibv1/Joints/Revolute  Orientation=down  DialogController=MECH.DynMechDlgSource  PhysicalDomain=mechanical  SubClassName=Unknown  LeftPortType=blob  RightPortType=blob  LConnTagsString=__newl0|SA1  RConnTagsString=__newr0  NumSAPorts=1  CutJoint=off  MarkAsCut=off  Primitives=revolute  PrimitiveProps=R1$WORLD$[0 0 1]$revolute  DialogClass=JointBlock  R1Axis=[0 0 1]
  B : PMIOPort  Orientation=down  Port=1  Side=Left
  F : PMIOPort  Orientation=up  Port=2  Side=Right
  wires:
  Constant/1 -> Mux/3, Mux/2
  Mux/1 -> Joint Actuator/1
  STEER/1 -> Mux/1
  connections:
  F/RConn1 -- Revolute/RConn1
  B/RConn1 -- Revolute/LConn1
  Joint Actuator/RConn1 -- Revolute/LConn2

== system mech_car_handling/FrontWheel2/WHEEL 1 ==
  FORCE : Inport  Orientation=left  OutDataType=sfix(16)  OutScaling=2^0
  Body : mblibv1/Bodies/Body  DialogController=MECH.DynMechDlgSource  PhysicalDomain=mechanical  SubClassName=Unknown  LeftPortType=workingframe  RightPortType=workingframe  LConnTagsString=CG  RConnTagsString=CS2|CS3  DialogClass=MechanicalBodyBlock  Mass=m  MassUnits=kg  InertiaUnits=kg*m^2  Inertia=I  Shape=Cylinder  ShapeDims=[1 1]  ShapeUnits=m  ShapeUse=false  Density=1  DensityUnits=kg/m^3  DensityUse=false  GraphicsMode=1  BodyColor=[0.5 0.5 0.5]  GraphicsObj=[]  AttachedToCS=1  CG=Left$CG$[0 0 0]$ADJOINING$ADJOINING$m$[0 0 0]$EULER X-Y-Z$deg$WORLD$true  WorkingFrames=Right$CS2$[0 0 -r]$CG$CG$m$[0 0 0]$EULER X-Y-Z$deg$WORLD$true#Left$CS1$[0 0 -r]$CG$CG$m$[0 0 0]$EULER X-Y-Z$deg$WORLD$false#Right$CS3$[0 0 -r]$CG$CG$m$[0 0 0]$EULER X-Y-Z$deg$WORLD$true  CGPos=[0 0 0]  CGRot=[0 0 0]  CS0Pos=[]  CS0Rot=[]  CS1Pos=[0 0 -r]  CS1Rot=[0 0 0]  CS2Pos=[0 0 -r]  CS2Rot=[0 0 0]  CS3Pos=[0 0 -r]  CS3Rot=[0 0 0]  CS4Pos=[]  CS4Rot=[]  CS5Pos=[]  CS5Rot=[]  CS6Pos=[]  CS6Rot=[]  CS7Pos=[]  CS7Rot=[]  CS8Pos=[]  CS8Rot=[]  CS9Pos=[]  CS9Rot=[]  CS10Pos=[]  CS10Rot=[]  CS11Pos=[]  CS11Rot=[]  CS12Pos=[]  CS12Rot=[]  CS13Pos=[]  CS13Rot=[]  CS14Pos=[]  CS14Rot=[]  CS15Pos=[]  CS15Rot=[]  CS16Pos=[]  CS16Rot=[]  CS17Pos=[]  CS17Rot=[]  CS18Pos=[]  CS18Rot=[]  CS19Pos=[]  CS19Rot=[]  CS20Pos=[]  CS20Rot=[]
  Body Actuator : mblibv1/Sensors &  Actuators/Body Actuator  Orientation=left  DialogController=MECH.DynMechDlgSource  SystemSampleTime=-1  PhysicalDomain=Mechanical  PortType=blob  ActuationStyle=Force  AngleUnits=deg  ArcVelocityUnits=deg/s  ArcAccelerationUnits=deg/s^2  CoordPositionUnits=m  VelocityUnits=m/s  AccelerationUnits=m/s^2  ForceUnits=N  TorqueUnits=N-m  ActiveIO=on  Width=3  DialogClass=MechanicalActuatorBlock  ReferenceFrame=Local (Body CS)  Angle=off  CoordPosition=on  Force=on  Torque=off
  Body Sensor : mblibv1/Sensors &  Actuators/Body Sensor  DialogController=MECH.DynMechDlgSource  SystemSampleTime=-1  PhysicalDomain=Mechanical  PortType=blob  Muxed=on  Pose=off  Angle=on  AngleUnits=deg  ArcVelocity=off  ArcVelocityUnits=deg/s  ArcAcceleration=off  ArcAccelerationUnits=deg/s^2  CoordPosition=off  CoordPositionUnits=m  Velocity=on  VelocityUnits=m/s  Acceleration=off  AccelerationUnits=m/s^2  Quaternion=on  QuaternionDT=off  QuaternionDDT=off  QuaternionUnits=off  OutputVector=[ 3 ]  ActiveIO=on  Width=3  DialogClass=MechanicalSensorBlock  ReferenceFrame=Local (Body CS)
  TO AXLE : PMIOPort  Port=1  Side=Left
  Sensed : Outport  OutDataType=sfix(16)  OutScaling=2^0
  wires:
  FORCE/1 -> Body Actuator/1
  Body Sensor/1 -> Sensed/1
  connections:
  Body Actuator/RConn1 -- Body/RConn2
  Body/RConn1 -- Body Sensor/LConn1
  TO AXLE/RConn1 -- Body/LConn1

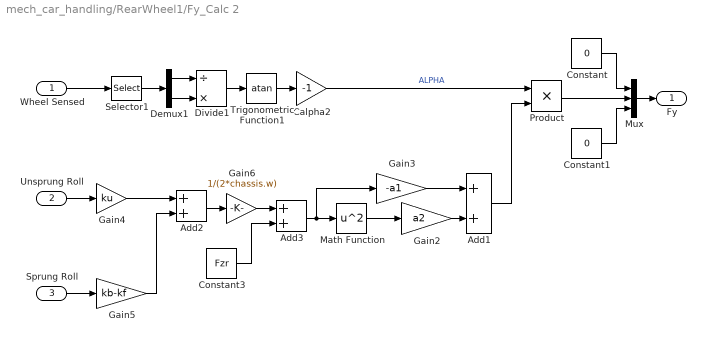
== system mech_car_handling/RearWheel1/Fy_Calc 2 ==
  Wheel Sensed : Inport  OutDataType=sfix(16)  OutScaling=2^0
  Unsprung Roll : Inport  Port=2  OutDataType=sfix(16)  OutScaling=2^0
  Sprung Roll : Inport  Port=3  OutDataType=sfix(16)  OutScaling=2^0
  Add1 : Sum  OutDataType=sfix(16)  OutScaling=2^-10
  Add2 : Sum  OutDataType=sfix(16)  OutScaling=2^-10
  Add3 : Sum  OutDataType=sfix(16)  OutScaling=2^-10
  Calpha2 : Gain  Gain=-1  ParameterDataType=sfix(16)  ParameterScaling=2^0  OutDataType=sfix(16)  OutScaling=2^0
  Constant : Constant  Value=0  OutDataType=sfix(16)  OutScaling=2^0
  Constant1 : Constant  Value=0  OutDataType=sfix(16)  OutScaling=2^0
  Constant3 : Constant  Value=Fzr  OutDataType=sfix(16)  OutScaling=2^0
  Demux1 : Demux  Outputs=2
  Divide1 : Product  Inputs=/*  OutDataType=sfix(16)  OutScaling=2^-10
  Gain2 : Gain  Gain=a2  ParameterDataType=sfix(16)  ParameterScaling=2^0  OutDataType=sfix(16)  OutScaling=2^0
  Gain3 : Gain  Gain=-a1  ParameterDataType=sfix(16)  ParameterScaling=2^0  OutDataType=sfix(16)  OutScaling=2^0
  Gain4 : Gain  Gain=ku  ParameterDataType=sfix(16)  ParameterScaling=2^0  OutDataType=sfix(16)  OutScaling=2^0
  Gain5 : Gain  Gain=kb-kf  ParameterDataType=sfix(16)  ParameterScaling=2^0  OutDataType=sfix(16)  OutScaling=2^0
  Gain6 : Gain  Gain=1/(2*chassis.w)  ParameterDataType=sfix(16)  ParameterScaling=2^0  OutDataType=sfix(16)  OutScaling=2^0
  Math Function : Math  Operator=square  OutDataType=sfix(16)  OutScaling=2^0  SaturateOnIntegerOverflow=on
  Mux : Mux  Inputs=3
  Product : Product  OutDataType=sfix(16)  OutScaling=2^0  RndMeth=Zero
  Selector1 : Selector  InputPortWidth=3  IndexOptions=Index vector (dialog)  Indices=[1 2]  OutputSizes=1
  Trigonometric Function1 : Trigonometry  Operator=atan
  Fy : Outport  OutDataType=sfix(16)  OutScaling=2^0
  wires:
  Calpha2/1 -> Product/1  "ALPHA"
  Divide1/1 -> Trigonometric Function1/1
  Demux1/2 -> Divide1/2
  Demux1/1 -> Divide1/1
  Selector1/1 -> Demux1/1
  Constant1/1 -> Mux/3
  Constant/1 -> Mux/1
  Mux/1 -> Fy/1
  Product/1 -> Mux/2
  Wheel Sensed/1 -> Selector1/1
  Trigonometric Function1/1 -> Calpha2/1
  Math Function/1 -> Gain2/1
  Gain2/1 -> Add1/2
  Gain3/1 -> Add1/1
  Add1/1 -> Product/2
  Unsprung Roll/1 -> Gain4/1
  Sprung Roll/1 -> Gain5/1
  Gain4/1 -> Add2/1
  Gain5/1 -> Add2/2
  Add2/1 -> Gain6/1
  Gain6/1 -> Add3/1
  Constant3/1 -> Add3/2
  Add3/1 -> Math Function/1, Gain3/1

== system mech_car_handling/RearWheel1/WHEEL 2 ==
  FORCE : Inport  Orientation=left  OutDataType=sfix(16)  OutScaling=2^0
  Body : mblibv1/Bodies/Body  DialogController=MECH.DynMechDlgSource  PhysicalDomain=mechanical  SubClassName=Unknown  LeftPortType=workingframe  RightPortType=workingframe  LConnTagsString=CG  RConnTagsString=CS2|CS3  DialogClass=MechanicalBodyBlock  Mass=m  MassUnits=kg  InertiaUnits=kg*m^2  Inertia=I  Shape=Cylinder  ShapeDims=[1 1]  ShapeUnits=m  ShapeUse=false  Density=1  DensityUnits=kg/m^3  DensityUse=false  GraphicsMode=1  BodyColor=[0.5 0.5 0.5]  GraphicsObj=[]  AttachedToCS=1  CG=Left$CG$[0 0 0]$ADJOINING$ADJOINING$m$[0 0 0]$EULER X-Y-Z$deg$WORLD$true  WorkingFrames=Right$CS2$[0 0 -r]$CG$CG$m$[0 0 0]$EULER X-Y-Z$deg$WORLD$true#Left$CS1$[0 0 -r]$CG$CG$m$[0 0 0]$EULER X-Y-Z$deg$WORLD$false#Right$CS3$[0 0 -r]$CG$CG$m$[0 0 0]$EULER X-Y-Z$deg$WORLD$true  CGPos=[0 0 0]  CGRot=[0 0 0]  CS0Pos=[]  CS0Rot=[]  CS1Pos=[0 0 -r]  CS1Rot=[0 0 0]  CS2Pos=[0 0 -r]  CS2Rot=[0 0 0]  CS3Pos=[0 0 -r]  CS3Rot=[0 0 0]  CS4Pos=[]  CS4Rot=[]  CS5Pos=[]  CS5Rot=[]  CS6Pos=[]  CS6Rot=[]  CS7Pos=[]  CS7Rot=[]  CS8Pos=[]  CS8Rot=[]  CS9Pos=[]  CS9Rot=[]  CS10Pos=[]  CS10Rot=[]  CS11Pos=[]  CS11Rot=[]  CS12Pos=[]  CS12Rot=[]  CS13Pos=[]  CS13Rot=[]  CS14Pos=[]  CS14Rot=[]  CS15Pos=[]  CS15Rot=[]  CS16Pos=[]  CS16Rot=[]  CS17Pos=[]  CS17Rot=[]  CS18Pos=[]  CS18Rot=[]  CS19Pos=[]  CS19Rot=[]  CS20Pos=[]  CS20Rot=[]
  Body Actuator : mblibv1/Sensors &  Actuators/Body Actuator  Orientation=left  DialogController=MECH.DynMechDlgSource  SystemSampleTime=-1  PhysicalDomain=Mechanical  PortType=blob  ActuationStyle=Force  AngleUnits=deg  ArcVelocityUnits=deg/s  ArcAccelerationUnits=deg/s^2  CoordPositionUnits=m  VelocityUnits=m/s  AccelerationUnits=m/s^2  ForceUnits=N  TorqueUnits=N-m  ActiveIO=on  Width=3  DialogClass=MechanicalActuatorBlock  ReferenceFrame=Local (Body CS)  Angle=off  CoordPosition=on  Force=on  Torque=off
  Body Sensor : mblibv1/Sensors &  Actuators/Body Sensor  DialogController=MECH.DynMechDlgSource  SystemSampleTime=-1  PhysicalDomain=Mechanical  PortType=blob  Muxed=on  Pose=off  Angle=on  AngleUnits=deg  ArcVelocity=off  ArcVelocityUnits=deg/s  ArcAcceleration=off  ArcAccelerationUnits=deg/s^2  CoordPosition=off  CoordPositionUnits=m  Velocity=on  VelocityUnits=m/s  Acceleration=off  AccelerationUnits=m/s^2  Quaternion=on  QuaternionDT=off  QuaternionDDT=off  QuaternionUnits=off  OutputVector=[ 3 ]  ActiveIO=on  Width=3  DialogClass=MechanicalSensorBlock  ReferenceFrame=Local (Body CS)
  TO AXLE : PMIOPort  Port=1  Side=Left
  Sensed : Outport  OutDataType=sfix(16)  OutScaling=2^0
  wires:
  Body Sensor/1 -> Sensed/1
  FORCE/1 -> Body Actuator/1
  connections:
  TO AXLE/RConn1 -- Body/LConn1
  Body/RConn1 -- Body Sensor/LConn1
  Body Actuator/RConn1 -- Body/RConn2

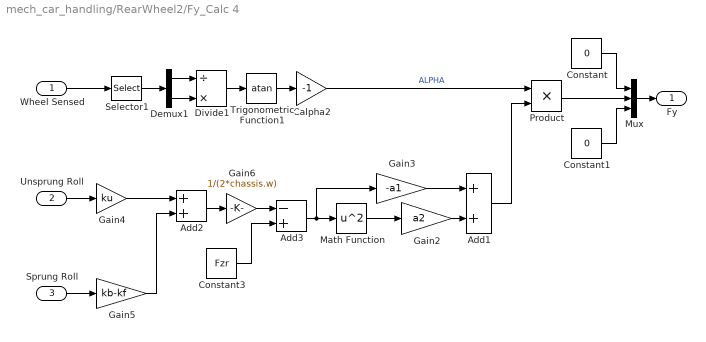
== system mech_car_handling/RearWheel2/Fy_Calc 4 ==
  Wheel Sensed : Inport  OutDataType=sfix(16)  OutScaling=2^0
  Unsprung Roll : Inport  Port=2  OutDataType=sfix(16)  OutScaling=2^0
  Sprung Roll : Inport  Port=3  OutDataType=sfix(16)  OutScaling=2^0
  Add1 : Sum  OutDataType=sfix(16)  OutScaling=2^-10
  Add2 : Sum  OutDataType=sfix(16)  OutScaling=2^-10
  Add3 : Sum  Inputs=-+  OutDataType=sfix(16)  OutScaling=2^-10
  Calpha2 : Gain  Gain=-1  ParameterDataType=sfix(16)  ParameterScaling=2^0  OutDataType=sfix(16)  OutScaling=2^0
  Constant : Constant  Value=0  OutDataType=sfix(16)  OutScaling=2^0
  Constant1 : Constant  Value=0  OutDataType=sfix(16)  OutScaling=2^0
  Constant3 : Constant  Value=Fzr  OutDataType=sfix(16)  OutScaling=2^0
  Demux1 : Demux  Outputs=2
  Divide1 : Product  Inputs=/*  OutDataType=sfix(16)  OutScaling=2^-10
  Gain2 : Gain  Gain=a2  ParameterDataType=sfix(16)  ParameterScaling=2^0  OutDataType=sfix(16)  OutScaling=2^0
  Gain3 : Gain  Gain=-a1  ParameterDataType=sfix(16)  ParameterScaling=2^0  OutDataType=sfix(16)  OutScaling=2^0
  Gain4 : Gain  Gain=ku  ParameterDataType=sfix(16)  ParameterScaling=2^0  OutDataType=sfix(16)  OutScaling=2^0
  Gain5 : Gain  Gain=kb-kf  ParameterDataType=sfix(16)  ParameterScaling=2^0  OutDataType=sfix(16)  OutScaling=2^0
  Gain6 : Gain  Gain=1/(2*chassis.w)  ParameterDataType=sfix(16)  ParameterScaling=2^0  OutDataType=sfix(16)  OutScaling=2^0
  Math Function : Math  Operator=square  OutDataType=sfix(16)  OutScaling=2^0  SaturateOnIntegerOverflow=on
  Mux : Mux  Inputs=3
  Product : Product  OutDataType=sfix(16)  OutScaling=2^0  RndMeth=Zero
  Selector1 : Selector  InputPortWidth=3  IndexOptions=Index vector (dialog)  Indices=[1 2]  OutputSizes=1
  Trigonometric Function1 : Trigonometry  Operator=atan
  Fy : Outport  OutDataType=sfix(16)  OutScaling=2^0
  wires:
  Add3/1 -> Gain3/1, Math Function/1
  Constant3/1 -> Add3/2
  Gain6/1 -> Add3/1
  Add2/1 -> Gain6/1
  Gain5/1 -> Add2/2
  Gain4/1 -> Add2/1
  Sprung Roll/1 -> Gain5/1
  Unsprung Roll/1 -> Gain4/1
  Add1/1 -> Product/2
  Gain3/1 -> Add1/1
  Gain2/1 -> Add1/2
  Math Function/1 -> Gain2/1
  Trigonometric Function1/1 -> Calpha2/1
  Wheel Sensed/1 -> Selector1/1
  Product/1 -> Mux/2
  Mux/1 -> Fy/1
  Constant/1 -> Mux/1
  Constant1/1 -> Mux/3
  Selector1/1 -> Demux1/1
  Demux1/1 -> Divide1/1
  Demux1/2 -> Divide1/2
  Divide1/1 -> Trigonometric Function1/1
  Calpha2/1 -> Product/1  "ALPHA"

== system mech_car_handling/RearWheel2/WHEEL 4 ==
  FORCE : Inport  Orientation=left  OutDataType=sfix(16)  OutScaling=2^0
  Body : mblibv1/Bodies/Body  DialogController=MECH.DynMechDlgSource  PhysicalDomain=mechanical  SubClassName=Unknown  LeftPortType=workingframe  RightPortType=workingframe  LConnTagsString=CG  RConnTagsString=CS2|CS3  DialogClass=MechanicalBodyBlock  Mass=m  MassUnits=kg  InertiaUnits=kg*m^2  Inertia=I  Shape=Cylinder  ShapeDims=[1 1]  ShapeUnits=m  ShapeUse=false  Density=1  DensityUnits=kg/m^3  DensityUse=false  GraphicsMode=1  BodyColor=[0.5 0.5 0.5]  GraphicsObj=[]  AttachedToCS=1  CG=Left$CG$[0 0 0]$ADJOINING$ADJOINING$m$[0 0 0]$EULER X-Y-Z$deg$WORLD$true  WorkingFrames=Right$CS2$[0 0 -r]$CG$CG$m$[0 0 0]$EULER X-Y-Z$deg$WORLD$true#Left$CS1$[0 0 -r]$CG$CG$m$[0 0 0]$EULER X-Y-Z$deg$WORLD$false#Right$CS3$[0 0 -r]$CG$CG$m$[0 0 0]$EULER X-Y-Z$deg$WORLD$true  CGPos=[0 0 0]  CGRot=[0 0 0]  CS0Pos=[]  CS0Rot=[]  CS1Pos=[0 0 -r]  CS1Rot=[0 0 0]  CS2Pos=[0 0 -r]  CS2Rot=[0 0 0]  CS3Pos=[0 0 -r]  CS3Rot=[0 0 0]  CS4Pos=[]  CS4Rot=[]  CS5Pos=[]  CS5Rot=[]  CS6Pos=[]  CS6Rot=[]  CS7Pos=[]  CS7Rot=[]  CS8Pos=[]  CS8Rot=[]  CS9Pos=[]  CS9Rot=[]  CS10Pos=[]  CS10Rot=[]  CS11Pos=[]  CS11Rot=[]  CS12Pos=[]  CS12Rot=[]  CS13Pos=[]  CS13Rot=[]  CS14Pos=[]  CS14Rot=[]  CS15Pos=[]  CS15Rot=[]  CS16Pos=[]  CS16Rot=[]  CS17Pos=[]  CS17Rot=[]  CS18Pos=[]  CS18Rot=[]  CS19Pos=[]  CS19Rot=[]  CS20Pos=[]  CS20Rot=[]
  Body Actuator : mblibv1/Sensors &  Actuators/Body Actuator  Orientation=left  DialogController=MECH.DynMechDlgSource  SystemSampleTime=-1  PhysicalDomain=Mechanical  PortType=blob  ActuationStyle=Force  AngleUnits=deg  ArcVelocityUnits=deg/s  ArcAccelerationUnits=deg/s^2  CoordPositionUnits=m  VelocityUnits=m/s  AccelerationUnits=m/s^2  ForceUnits=N  TorqueUnits=N-m  ActiveIO=on  Width=3  DialogClass=MechanicalActuatorBlock  ReferenceFrame=Local (Body CS)  Angle=off  CoordPosition=on  Force=on  Torque=off
  Body Sensor : mblibv1/Sensors &  Actuators/Body Sensor  DialogController=MECH.DynMechDlgSource  SystemSampleTime=-1  PhysicalDomain=Mechanical  PortType=blob  Muxed=on  Pose=off  Angle=on  AngleUnits=deg  ArcVelocity=off  ArcVelocityUnits=deg/s  ArcAcceleration=off  ArcAccelerationUnits=deg/s^2  CoordPosition=off  CoordPositionUnits=m  Velocity=on  VelocityUnits=m/s  Acceleration=off  AccelerationUnits=m/s^2  Quaternion=on  QuaternionDT=off  QuaternionDDT=off  QuaternionUnits=off  OutputVector=[ 3 ]  ActiveIO=on  Width=3  DialogClass=MechanicalSensorBlock  ReferenceFrame=Local (Body CS)
  TO AXLE : PMIOPort  Port=1  Side=Left
  Sensed : Outport  OutDataType=sfix(16)  OutScaling=2^0
  wires:
  FORCE/1 -> Body Actuator/1
  Body Sensor/1 -> Sensed/1
  connections:
  Body Actuator/RConn1 -- Body/RConn2
  Body/RConn1 -- Body Sensor/LConn1
  TO AXLE/RConn1 -- Body/LConn1

== system mech_car_handling/Sprung System/SPRUNG MASS ==
  Body : mblibv1/Bodies/Body  DialogController=MECH.DynMechDlgSource  PhysicalDomain=mechanical  SubClassName=Unknown  LeftPortType=workingframe  RightPortType=workingframe  LConnTagsString=CG  RConnTagsString=CS3  DialogClass=MechanicalBodyBlock  Mass=m  MassUnits=kg  InertiaUnits=kg*m^2  Inertia=eye(3)  Shape=Cylinder  ShapeDims=[1 1]  ShapeUnits=m  ShapeUse=false  Density=1  DensityUnits=kg/m^3  DensityUse=false  GraphicsMode=1  BodyColor=[0.5 0.5 0.5]  GraphicsObj=[]  AttachedToCS=1  CG=Left$CG$[0 0 h]$CS3$CS3$m$[0 0 0]$Euler X-Y-Z$deg$WORLD$true  WorkingFrames=Right$CS1$[0 0 0]$CG$CG$m$[0 0 0]$Euler X-Y-Z$deg$WORLD$false#Right$CS3$[0 0 0]$ADJOINING$ADJOINING$m$[0 0 0]$Euler X-Y-Z$deg$WORLD$true  CGPos=[0 0 h]  CGRot=[0 0 0]  CS0Pos=[]  CS0Rot=[]  CS1Pos=[0 0 0]  CS1Rot=[0 0 0]  CS2Pos=[]  CS2Rot=[]  CS3Pos=[0 0 0]  CS3Rot=[0 0 0]  CS4Pos=[]  CS4Rot=[]  CS5Pos=[]  CS5Rot=[]  CS6Pos=[]  CS6Rot=[]  CS7Pos=[]  CS7Rot=[]  CS8Pos=[]  CS8Rot=[]  CS9Pos=[]  CS9Rot=[]  CS10Pos=[]  CS10Rot=[]  CS11Pos=[]  CS11Rot=[]  CS12Pos=[]  CS12Rot=[]  CS13Pos=[]  CS13Rot=[]  CS14Pos=[]  CS14Rot=[]  CS15Pos=[]  CS15Rot=[]  CS16Pos=[]  CS16Rot=[]  CS17Pos=[]  CS17Rot=[]  CS18Pos=[]  CS18Rot=[]  CS19Pos=[]  CS19Rot=[]  CS20Pos=[]  CS20Rot=[]
  TO M UNSPRUNG : PMIOPort  Orientation=left  Port=1  Side=Right
  connections:
  Body/RConn1 -- TO M UNSPRUNG/RConn1

== system mech_car_handling/Sprung System/TORSIONAL SPRING1 ==
  Joint Sensor : mblibv1/Sensors &  Actuators/Joint Sensor  DialogController=MECH.DynMechDlgSource  SystemSampleTime=-1  PhysicalDomain=Mechanical  PortType=blob  Muxed=on  Pose=off  Angle=on  AngleUnits=rad  ArcVelocity=off  ArcVelocityUnits=deg/s  ArcAcceleration=off  ArcAccelerationUnits=deg/s^2  CoordPosition=on  CoordPositionUnits=m  Velocity=off  VelocityUnits=m/s  Acceleration=off  AccelerationUnits=m/s^2  Quaternion=on  QuaternionDT=off  QuaternionDDT=off  QuaternionUnits=off  OutputVector=[ 1 ]  ActiveIO=on  Width=1  DialogClass=MechanicalSensorBlock  Primitive=R1  Force=off  ForceUnits=N  Torque=off  TorqueUnits=N-m  ReferenceFrame=Absolute (INERTIAL)  ReactionSensedSide=Base  ReactionReferenceFrame=Local (Body CS)  ReactionForce=off  ReactionForceUnits=N  ReactionMoment=off  ReactionMomentUnits=N-m
  Joint Spring & Damper : mblibv1/Force  Elements/Joint Spring & Damper  Orientation=left  DialogController=MECH.DynMechDlgSource  SystemSampleTime=-1  DialogClass=JointSpringDamper  JFEParameters=P1$false$0$0$0$m$m/s$N$rad$rad/s$N-m#P2$false$0$0$0$m$m/s$N$rad$rad/s$N-m#P3$false$0$0$0$m$m/s$N$rad$rad/s$N-m#R1$true$kr$br$0$m$m/s$N$rad$rad/s$N-m#R2$false$0$0$0$m$m/s$N$rad$rad/s$N-m#R3$false$0$0$0$m$m/s$N$rad$rad/s$N-m#S$false$0$0$0$m$m/s$N$rad$rad/s$N-m
  Revolute : mblibv1/Joints/Revolute  DialogController=MECH.DynMechDlgSource  PhysicalDomain=mechanical  SubClassName=Unknown  LeftPortType=blob  RightPortType=blob  LConnTagsString=__newl0|SA1  RConnTagsString=__newr0|SA1  NumSAPorts=2  CutJoint=off  MarkAsCut=off  Primitives=revolute  PrimitiveProps=R1$Base$[1 0 0]$revolute  DialogClass=JointBlock  R1Axis=[1 0 0]
  B : PMIOPort  Port=1  Side=Left
  F : PMIOPort  Orientation=left  Port=2  Side=Right
  Roll : Outport  OutDataType=sfix(16)  OutScaling=2^0
  wires:
  Joint Sensor/1 -> Roll/1
  connections:
  F/RConn1 -- Revolute/RConn1
  B/RConn1 -- Revolute/LConn1
  Joint Spring & Damper/LConn1 -- Revolute/LConn2
  Joint Sensor/LConn1 -- Revolute/RConn2

== system mech_car_handling/Unsprung System/TORSIONAL SPRING ==
  Joint Sensor : mblibv1/Sensors &  Actuators/Joint Sensor  DialogController=MECH.DynMechDlgSource  SystemSampleTime=-1  PhysicalDomain=Mechanical  PortType=blob  Muxed=on  Pose=off  Angle=on  AngleUnits=rad  ArcVelocity=off  ArcVelocityUnits=deg/s  ArcAcceleration=off  ArcAccelerationUnits=deg/s^2  CoordPosition=on  CoordPositionUnits=m  Velocity=off  VelocityUnits=m/s  Acceleration=off  AccelerationUnits=m/s^2  Quaternion=on  QuaternionDT=off  QuaternionDDT=off  QuaternionUnits=off  OutputVector=[ 1 ]  ActiveIO=on  Width=1  DialogClass=MechanicalSensorBlock  Primitive=R1  Force=off  ForceUnits=N  Torque=off  TorqueUnits=N-m  ReferenceFrame=Absolute (INERTIAL)  ReactionSensedSide=Base  ReactionReferenceFrame=Local (Body CS)  ReactionForce=off  ReactionForceUnits=N  ReactionMoment=off  ReactionMomentUnits=N-m
  Joint Spring & Damper : mblibv1/Force  Elements/Joint Spring & Damper  Orientation=left  DialogController=MECH.DynMechDlgSource  SystemSampleTime=-1  DialogClass=JointSpringDamper  JFEParameters=P1$false$0$0$0$m$m/s$N$rad$rad/s$N-m#P2$false$0$0$0$m$m/s$N$rad$rad/s$N-m#P3$false$0$0$0$m$m/s$N$rad$rad/s$N-m#R1$true$ku$bu$0$m$m/s$N$rad$rad/s$N-m#R2$false$0$0$0$m$m/s$N$rad$rad/s$N-m#R3$false$0$0$0$m$m/s$N$rad$rad/s$N-m#S$false$0$0$0$m$m/s$N$rad$rad/s$N-m
  Revolute : mblibv1/Joints/Revolute  DialogController=MECH.DynMechDlgSource  PhysicalDomain=mechanical  SubClassName=Unknown  LeftPortType=blob  RightPortType=blob  LConnTagsString=__newl0|SA1  RConnTagsString=__newr0|SA1  NumSAPorts=2  CutJoint=off  MarkAsCut=off  Primitives=revolute  PrimitiveProps=R1$Base$[1 0 0]$revolute  DialogClass=JointBlock  R1Axis=[1 0 0]
  B : PMIOPort  Port=1  Side=Left
  F : PMIOPort  Orientation=left  Port=2  Side=Right
  Roll : Outport  OutDataType=sfix(16)  OutScaling=2^0
  wires:
  Joint Sensor/1 -> Roll/1
  connections:
  Joint Sensor/LConn1 -- Revolute/RConn2
  Joint Spring & Damper/LConn1 -- Revolute/LConn2
  B/RConn1 -- Revolute/LConn1
  F/RConn1 -- Revolute/RConn1
